simulink model "model_2"  (R2021b)
settings: Solver=VariableStepAuto  StartTime=0.0  StopTime=50  RelTol=1e-3
undefined symbols (not defined in the file): k
settings Model: Creator=vital  LastModifiedBy=vital

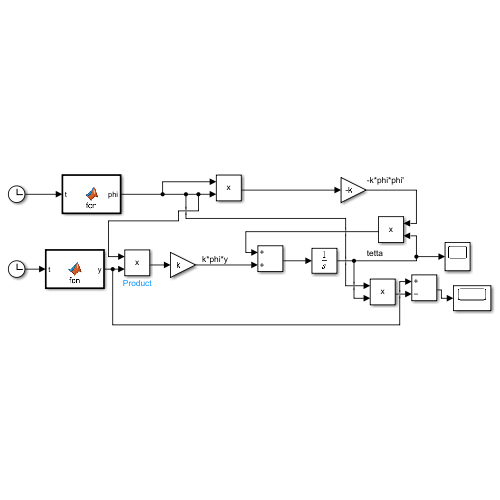
[thumbnail: Simulink's stored preview of the top-level diagram]
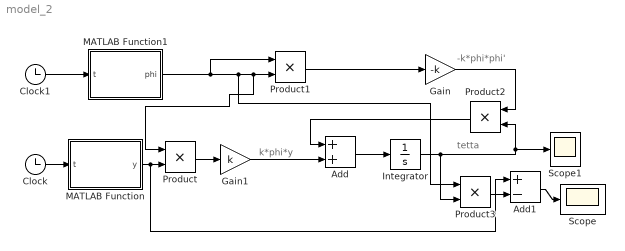
== system model_2 ==
  note: tetta
  note: -k*phi*phi'
  note: k*phi*y
  Add : Sum
  Add1 : Sum  Inputs=+-
  Clock : Clock
  Clock1 : Clock
  Gain : Gain  Gain=-k
  Gain1 : Gain  Gain=k
  Integrator : Integrator
  MATLAB Function : MATLAB Function  TreatAsAtomicUnit=on
  MATLAB Function1 : MATLAB Function  TreatAsAtomicUnit=on
  Product{,1..3} (4 alike) : Product
  Scope : Scope
  Scope1 : Scope
  wires:
  Product3/1 -> Add1/2
  MATLAB Function1/1(phi) -> Product1/1, Product3/1, Product1/2, Product/1
  Add/1 -> Integrator/1
  MATLAB Function/1(y) -> Add1/1, Product/2
  Product2/1 -> Add/1
  Gain1/1 -> Add/2
  Integrator/1 -> Product3/2, Scope1/1, Product2/2
  Clock1/1 -> MATLAB Function1/1(t)
  Product/1 -> Gain1/1
  Clock/1 -> MATLAB Function/1(t)
  Gain/1 -> Product2/1
  Add1/1 -> Scope/1
  Product1/1 -> Gain/1

== matlab function model_2/MATLAB Function ==
  data: t input; y output
function y = fcn(t)

y = 10*cos(t+pi/3);

== matlab function model_2/MATLAB Function1 ==
  data: t input; phi output
function phi = fcn(t)

phi = t;
